simulink model "timeline"  (Simulink 7.5)
settings: Solver=FixedStepDiscrete  StartTime=0.0  StopTime=inf  FixedStep=.5  RelTol=1e-3
libraries: nxt_Lib x18, Nokia_Arduino_Blocks x4
settings Model: Creator=tyler  LastModifiedBy=Wildcat
settings DebuggingCC: MultiTaskDSMMsg=none  StrictBusMsg=Warning
settings HardwareCC: ProdEndianess=LittleEndian  ProdHWDeviceType=ARM Compatible->ARM 7
settings RTWCC: SystemTargetFile=nrt.tlc  GenCodeOnly=on  TemplateMakefile=nrt_unix.tmf  Description=Nokia Real-Time Target  ProcessScript=nrt_make_rtw_hook
settings STFCustomTargetCC: ModelReferenceCompliant=off  GeneratePreprocessorConditionals=Disable all  MatFileLogging=on  SystemTargetFile=nrt.tlc
settings GRTTargetCC: ModelReferenceCompliant=off  ParMdlRefBuildCompliant=off  CompOptLevelCompliant=off
settings CustomProperty: DataType=string  Value=-lm -ldl
settings EnumStrPairs: String=PC

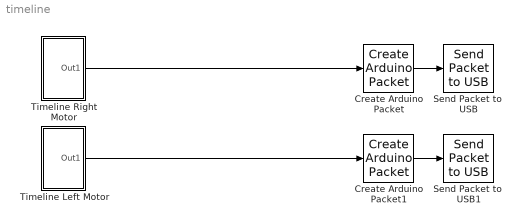
== system timeline ==
  Create Arduino Packet : Nokia_Arduino_Blocks/Create Arduino Packet  SystemSampleTime=-1  rOrW=Write  command=Motor  numPort=1
  Create Arduino Packet1 : Nokia_Arduino_Blocks/Create Arduino Packet  SystemSampleTime=-1  rOrW=Write  command=Motor  numPort=2
  Send Packet to  USB : Nokia_Arduino_Blocks/Send Packet to  USB
  Send Packet to  USB1 : Nokia_Arduino_Blocks/Send Packet to  USB
  Timeline Left Motor : Subsystem
  Timeline Right Motor : Subsystem
  wires:
  Timeline Right Motor/1(Out1) -> Create Arduino Packet/1
  Create Arduino Packet/1 -> Send Packet to  USB/1
  Create Arduino Packet1/1 -> Send Packet to  USB1/1
  Timeline Left Motor/1(Out1) -> Create Arduino Packet1/1

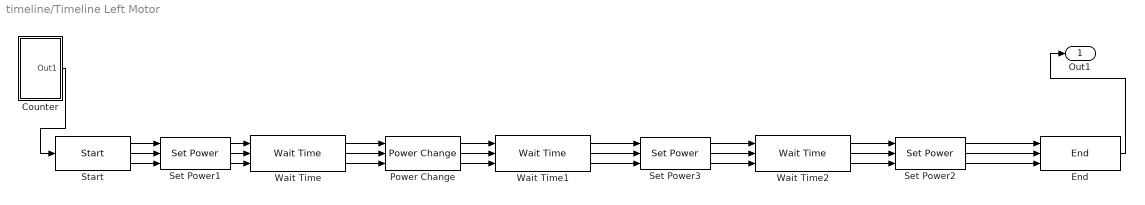
== system timeline/Timeline Left Motor ==
  Counter : Subsystem
  End : nxt_Lib/End  SystemSampleTime=-1
  Power Change : nxt_Lib/Power Change  SystemSampleTime=-1  c=-255
  Set Power1 : nxt_Lib/Set Power  SystemSampleTime=-1  a=512
  Set Power2 : nxt_Lib/Set Power  SystemSampleTime=-1  a=255
  Set Power3 : nxt_Lib/Set Power  SystemSampleTime=-1  a=512
  Start : nxt_Lib/Start  SystemSampleTime=-1
  Wait Time : nxt_Lib/Wait Time  SystemSampleTime=-1  b=4
  Wait Time1 : nxt_Lib/Wait Time  SystemSampleTime=-1  b=1
  Wait Time2 : nxt_Lib/Wait Time  SystemSampleTime=-1  b=3
  Out1 : Outport
  wires:
  Start/1 -> Set Power1/1
  Start/2 -> Set Power1/2
  Set Power1/1 -> Wait Time/1
  Set Power1/2 -> Wait Time/2
  Wait Time/1 -> Power Change/1
  Wait Time/2 -> Power Change/2
  Power Change/1 -> Wait Time1/1
  Power Change/2 -> Wait Time1/2
  Wait Time1/1 -> Set Power3/1
  Wait Time1/2 -> Set Power3/2
  Set Power3/1 -> Wait Time2/1
  End/1 -> Out1/1
  Set Power1/3 -> Wait Time/3
  Start/3 -> Set Power1/3
  Wait Time/3 -> Power Change/3
  Power Change/3 -> Wait Time1/3
  Wait Time1/3 -> Set Power3/3
  Set Power3/2 -> Wait Time2/2
  Set Power3/3 -> Wait Time2/3
  Set Power2/1 -> End/1
  Set Power2/2 -> End/2
  Set Power2/3 -> End/3
  Wait Time2/1 -> Set Power2/1
  Wait Time2/2 -> Set Power2/2
  Wait Time2/3 -> Set Power2/3
  Counter/1(Out1) -> Start/1

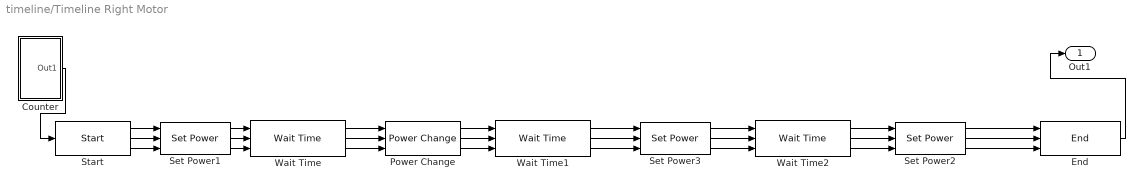
== system timeline/Timeline Right Motor ==
  Counter : Subsystem
  End : nxt_Lib/End  SystemSampleTime=-1
  Power Change : nxt_Lib/Power Change  SystemSampleTime=-1  c=-100
  Set Power1 : nxt_Lib/Set Power  SystemSampleTime=-1  a=512
  Set Power2 : nxt_Lib/Set Power  SystemSampleTime=-1  a=255
  Set Power3 : nxt_Lib/Set Power  SystemSampleTime=-1  a=512
  Start : nxt_Lib/Start  SystemSampleTime=-1
  Wait Time : nxt_Lib/Wait Time  SystemSampleTime=-1  b=4
  Wait Time1 : nxt_Lib/Wait Time  SystemSampleTime=-1  b=1
  Wait Time2 : nxt_Lib/Wait Time  SystemSampleTime=-1  b=3
  Out1 : Outport
  wires:
  Start/1 -> Set Power1/1
  Start/2 -> Set Power1/2
  Set Power1/1 -> Wait Time/1
  Set Power1/2 -> Wait Time/2
  Wait Time/1 -> Power Change/1
  Wait Time/2 -> Power Change/2
  Power Change/1 -> Wait Time1/1
  Power Change/2 -> Wait Time1/2
  Wait Time1/1 -> Set Power3/1
  Wait Time1/2 -> Set Power3/2
  Set Power3/1 -> Wait Time2/1
  End/1 -> Out1/1
  Set Power1/3 -> Wait Time/3
  Start/3 -> Set Power1/3
  Wait Time/3 -> Power Change/3
  Power Change/3 -> Wait Time1/3
  Wait Time1/3 -> Set Power3/3
  Set Power3/2 -> Wait Time2/2
  Set Power3/3 -> Wait Time2/3
  Set Power2/1 -> End/1
  Set Power2/2 -> End/2
  Set Power2/3 -> End/3
  Wait Time2/1 -> Set Power2/1
  Wait Time2/2 -> Set Power2/2
  Wait Time2/3 -> Set Power2/3
  Counter/1(Out1) -> Start/1

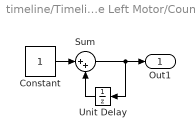
== system timeline/Timeline Left Motor/Counter ==
  Constant : Constant  OutDataType=fixdt(1, 16)  OutScaling=2^0
  Sum : Sum  Inputs=|++  OutDataType=fixdt(1, 16)  OutScaling=2^0
  Unit Delay : UnitDelay  SampleTime=-1
  Out1 : Outport
  wires:
  Sum/1 -> Unit Delay/1, Out1/1
  Unit Delay/1 -> Sum/2
  Constant/1 -> Sum/1

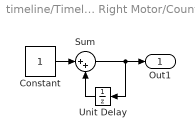
== system timeline/Timeline Right Motor/Counter ==
  Constant : Constant  OutDataType=fixdt(1, 16)  OutScaling=2^0
  Sum : Sum  Inputs=|++  OutDataType=fixdt(1, 16)  OutScaling=2^0
  Unit Delay : UnitDelay  SampleTime=-1
  Out1 : Outport
  wires:
  Sum/1 -> Unit Delay/1, Out1/1
  Unit Delay/1 -> Sum/2
  Constant/1 -> Sum/1
